simulink model "generic_IVS"  (R2024a)
settings: Solver=FixedStepDiscrete  StartTime=0.0  StopTime=inf  FixedStep=0.001  RelTol=1e-3
undefined symbols (not defined in the file): do_waypoints_tail_shifted_2, pathXY, route1_waypoint, route1_waypoint_raw, route2_waypoint, route2_waypoint_raw, route3_waypoint, route3_waypoint_raw, waypoints2
libraries: CarMaker4SL x431, slpidlib x19, dspsigops x3, simulink x1
(part 2 of 15)

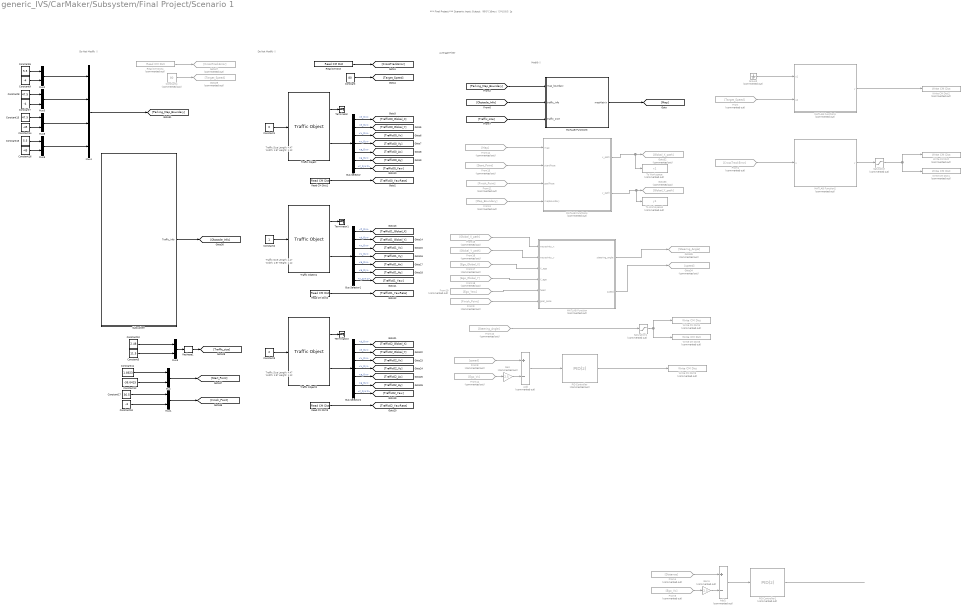
== system generic_IVS/CarMaker/Subsystem/Final Project/Scenario 1 ==
  note: Do Not Modify !!
  note: Traffic Size
      | Length: 4.47
      | Width: 1.97
      | Height: 1.12
  note: Traffic Size
      | Length: 4.47
      | Width: 1.97
      | Height: 1.12
  note: Traffic Size
      | Length: 4.47
      | Width: 1.97
      | Height: 1.12
  note: *** Final Project ***
      |
      | Scenario:
      | Input:
      | Output:
      | 제어기 10ms / 다익스트라 1s
  note: Do Not Modify !!
  note: Modify !!
  note: Average Filter
  Add : Sum  Commented=on  Inputs=+-
  Add1 : Sum  Commented=on  Inputs=+-
  Bus Selector : BusSelector  OutputSignals=t_0 x,t_0 y,v_0 x,v_0 y,a_0 x,a_0 y,r_zyx z
  Bus Selector1 : BusSelector  OutputSignals=t_0 x,t_0 y,v_0 x,v_0 y,a_0 x,a_0 y,r_zyx z
  Bus Selector2 : BusSelector  OutputSignals=t_0 x,t_0 y,v_0 x,v_0 y,a_0 x,a_0 y,r_zyx z
  Constant : Constant  Value=80
  Constant1 : Constant  Value=0
  Constant10 : Constant  Value=2.48
  Constant11 : Constant  Value=1.8923
  Constant12 : Constant  Value=-36.6415
  Constant13 : Constant  Value=47.5
  Constant14 : Constant  Value=-45
  Constant15 : Constant  Value=5.5
  Constant16 : Constant  Value=-45
  Constant17 : Constant  Value=36.5
  Constant18 : Constant  Value=-3
  Constant2 : Constant
  Constant3 : Constant  Value=2
  Constant4 : Constant  Commented=on  Value=80
  Constant5 : Constant  Value=11.5
  Constant6 : Constant  Value=5.5
  Constant7 : Constant  Value=-4
  Constant8 : Constant  Value=47.5
  Constant9 : Constant  Value=-4
  From : From  Commented=on  GotoTag=Target_Speed
  From1 : From  Commented=on  GotoTag=CrossTrackError
  From10 : From  Commented=on  GotoTag=Steering_Angle
  From11 : From  Commented=on  GotoTag=Finish_Point
  From12 : From  Commented=on  GotoTag=Map
  From13 : From  Commented=on  GotoTag=Start_Point
  From14 : From  Commented=on  GotoTag=Ego_Vx
  From15 : From  Commented=on  GotoTag=Global_X_path
  From16 : From  Commented=on  GotoTag=Global_Y_path
  From17 : From  Commented=on  GotoTag=Ego_Global_X
  From18 : From  Commented=on  GotoTag=Ego_Global_Y
  From19 : From  Commented=on  GotoTag=Ego_Yaw
  From3 : From  Commented=on  GotoTag=Map_Boundary
  From4 : From  Commented=on  GotoTag=Distance
  From5 : From  Commented=on  GotoTag=Ego_Vx
  From8 : From  Commented=on  GotoTag=speed
  From9 : From  Commented=on  GotoTag=Finish_Point
  Gain : Gain  Commented=on  Gain=2.5
  Gain1 : Gain  Commented=on  Gain=2.5
  Goto27 : Goto  Commented=on  GotoTag=CrossTrackError
  Goto29 : Goto  Commented=on  GotoTag=Target_Speed
  Goto32 : Goto  Commented=on  GotoTag=Global_X_path
  Goto33 : Goto  Commented=on  GotoTag=Global_Y_path
  Goto34 : Goto  Commented=on  GotoTag=speed
  Goto35 : Goto  Commented=on  GotoTag=Steering_Angle
  Ground : Ground  Commented=on
  MATLAB Function : MATLAB Function  Commented=on  TreatAsAtomicUnit=on
  MATLAB Function1 : MATLAB Function  Commented=on  TreatAsAtomicUnit=on
  MATLAB Function2 : MATLAB Function  Commented=on  TreatAsAtomicUnit=on
  MATLAB Function3 : MATLAB Function  TreatAsAtomicUnit=on
  MATLAB Function4 : MATLAB Function  Commented=on  TreatAsAtomicUnit=on
  Mux{,1..3,5,8..9} (7 alike) : Mux  Inputs=2
  Mux4 : Mux
  PID Controller : slpidlib/PID Controller  Commented=on  Controller=PID  Form=Parallel  TimeDomain=Discrete-time  UseExternalTs=off  SampleTime=-1  IntegratorMethod=Forward Euler  FilterMethod=Forward Euler  ControllerParametersSource=internal  P=1  I=0  UseKiTs=off  D=0  UseExternalDerivativeSource=off  N=100  UseFilter=off  TunerSelectOption=Transfer Function Based (PID Tuner App)  InitialConditionSource=internal  InitialConditionForIntegrator=0  InitialConditionForFilter=0  DifferentiatorICPrevScaledInput=0  ExternalReset=none  TrackingMode=off  Kt=1  LimitOutput=off  SatLimitsSource=internal  UpperSaturationLimit=inf  LowerSaturationLimit=-inf  LinearizeAsGain=on  AntiWindupMode=none  Kb=1  LimitIntegrator=off  UpperIntegratorSaturationLimit=inf  LowerIntegratorSaturationLimit=-inf  POutMin=[]  POutMax=[]  IOutMin=[]  IOutMax=[]  DOutMin=[]  DOutMax=[]  NOutMin=[]  NOutMax=[]  SumOutMin=[]  SumOutMax=[]  SaturationOutMin=[]  SaturationOutMax=[]  PParamMin=[]  PParamMax=[]  IParamMin=[]  IParamMax=[]  DParamMin=[]  DParamMax=[]  NParamMin=[]  NParamMax=[]  KbParamMin=[]  KbParamMax=[]  KtParamMin=[]  KtParamMax=[]  KbOutMin=[]  KbOutMax=[]  KtOutMin=[]  KtOutMax=[]  IntegratorOutMin=[]  IntegratorOutMax=[]  FilterOutMin=[]  FilterOutMax=[]  SumI1OutMin=[]  SumI1OutMax=[]  SumI2OutMin=[]  SumI2OutMax=[]  SumI3OutMin=[]  SumI3OutMax=[]  SumI4OutMin=[]  SumI4OutMax=[]  SumDOutMin=[]  SumDOutMax=[]  DifferentiatorOutMin=[]  DifferentiatorOutMax=[]  FilterDiffOutCoefMin=[]  FilterDiffOutCoefMax=[]  ReciprocalOutMin=[]  ReciprocalOutMax=[]  SumDenOutMin=[]  SumDenOutMax=[]  SumNumOutMin=[]  SumNumOutMax=[]  DivideOutMin=[]  DivideOutMax=[]  UdiffTsProdOutMin=[]  UdiffTsProdOutMax=[]  NTsProdOutMin=[]  NTsProdOutMax=[]  UintegralTsProdOutMin=[]  UintegralTsProdOutMax=[]  UngainTsProdOutMin=[]  UngainTsProdOutMax=[]  ClampingZeroOutDataTypeStr=Inherit: Inherit via back propagation  ClampingZeroOutMin=[]  ClampingZeroOutMax=[]  FilterDenConstantOutDataTypeStr=Inherit: Inherit via back propagation  FilterDenConstantOutMin=[]  FilterDenConstantOutMax=[]  PCopyOutDataTypeStr=Inherit: Inherit via back propagation  PCopyOutMin=[]  PCopyOutMax=[]  NCopyOutDataTypeStr=Inherit: Inherit via back propagation  NCopyOutMin=[]  NCopyOutMax=[]  IntegratorContinuousStateAttributes=''  IntegratorStateMustResolveToSignalObject=off  IntegratorRTWStateStorageClass=Auto  FilterContinuousStateAttributes=''  FilterStateMustResolveToSignalObject=off  FilterRTWStateStorageClass=Auto  ParallelPVariant=InternalParameters  IdealPVariant=Disabled  IVariant=InternalParameters  DVariant=InternalParameters  IntegratorVariant=Discrete  SatVariant=Disabled  AWVariant=Passthrough  PCopyVariant=Disabled  TRVariant=Disabled  FdbkBlocksVariant=Forward  IdealPFdbkVariant=Disabled  SatFdbkVariant=Disabled  DerivativeFilterVariant=Differentiator  NVariant=Passthrough  NCopyVariant=Disabled_SignalSpec  FilterICVariant=InternalICsDifferentiator  IntegratorICVariant=InternalICs  ExternalResetVariant=Disabled  TRSumVariant=Passthrough  SumFdbkVariant=Disabled  SumVariant=Sum_PID  TsampFilterVariant=InternalTs  TsampNgainVariant=Passthrough  TsampIntegralVariant=Disabled_SignalSpec  ExternalSaturationOutDataTypeStr=Inherit: Same as second input  DerivativeSourceVariant=ErrorSignal
  PID Controller1 : slpidlib/PID Controller  Commented=on  Controller=PID  Form=Parallel  TimeDomain=Discrete-time  UseExternalTs=off  SampleTime=-1  IntegratorMethod=Forward Euler  FilterMethod=Forward Euler  ControllerParametersSource=internal  P=5  I=0  UseKiTs=off  D=0  UseExternalDerivativeSource=off  N=100  UseFilter=off  TunerSelectOption=Transfer Function Based (PID Tuner App)  InitialConditionSource=internal  InitialConditionForIntegrator=0  InitialConditionForFilter=0  DifferentiatorICPrevScaledInput=0  ExternalReset=none  TrackingMode=off  Kt=1  LimitOutput=off  SatLimitsSource=internal  UpperSaturationLimit=inf  LowerSaturationLimit=-inf  LinearizeAsGain=on  AntiWindupMode=none  Kb=1  LimitIntegrator=off  UpperIntegratorSaturationLimit=inf  LowerIntegratorSaturationLimit=-inf  POutMin=[]  POutMax=[]  IOutMin=[]  IOutMax=[]  DOutMin=[]  DOutMax=[]  NOutMin=[]  NOutMax=[]  SumOutMin=[]  SumOutMax=[]  SaturationOutMin=[]  SaturationOutMax=[]  PParamMin=[]  PParamMax=[]  IParamMin=[]  IParamMax=[]  DParamMin=[]  DParamMax=[]  NParamMin=[]  NParamMax=[]  KbParamMin=[]  KbParamMax=[]  KtParamMin=[]  KtParamMax=[]  KbOutMin=[]  KbOutMax=[]  KtOutMin=[]  KtOutMax=[]  IntegratorOutMin=[]  IntegratorOutMax=[]  FilterOutMin=[]  FilterOutMax=[]  SumI1OutMin=[]  SumI1OutMax=[]  SumI2OutMin=[]  SumI2OutMax=[]  SumI3OutMin=[]  SumI3OutMax=[]  SumI4OutMin=[]  SumI4OutMax=[]  SumDOutMin=[]  SumDOutMax=[]  DifferentiatorOutMin=[]  DifferentiatorOutMax=[]  FilterDiffOutCoefMin=[]  FilterDiffOutCoefMax=[]  ReciprocalOutMin=[]  ReciprocalOutMax=[]  SumDenOutMin=[]  SumDenOutMax=[]  SumNumOutMin=[]  SumNumOutMax=[]  DivideOutMin=[]  DivideOutMax=[]  UdiffTsProdOutMin=[]  UdiffTsProdOutMax=[]  NTsProdOutMin=[]  NTsProdOutMax=[]  UintegralTsProdOutMin=[]  UintegralTsProdOutMax=[]  UngainTsProdOutMin=[]  UngainTsProdOutMax=[]  ClampingZeroOutDataTypeStr=Inherit: Inherit via back propagation  ClampingZeroOutMin=[]  ClampingZeroOutMax=[]  FilterDenConstantOutDataTypeStr=Inherit: Inherit via back propagation  FilterDenConstantOutMin=[]  FilterDenConstantOutMax=[]  PCopyOutDataTypeStr=Inherit: Inherit via back propagation  PCopyOutMin=[]  PCopyOutMax=[]  NCopyOutDataTypeStr=Inherit: Inherit via back propagation  NCopyOutMin=[]  NCopyOutMax=[]  IntegratorContinuousStateAttributes=''  IntegratorStateMustResolveToSignalObject=off  IntegratorRTWStateStorageClass=Auto  FilterContinuousStateAttributes=''  FilterStateMustResolveToSignalObject=off  FilterRTWStateStorageClass=Auto  ParallelPVariant=InternalParameters  IdealPVariant=Disabled  IVariant=InternalParameters  DVariant=InternalParameters  IntegratorVariant=Discrete  SatVariant=Disabled  AWVariant=Passthrough  PCopyVariant=Disabled  TRVariant=Disabled  FdbkBlocksVariant=Forward  IdealPFdbkVariant=Disabled  SatFdbkVariant=Disabled  DerivativeFilterVariant=Differentiator  NVariant=Passthrough  NCopyVariant=Disabled_SignalSpec  FilterICVariant=InternalICsDifferentiator  IntegratorICVariant=InternalICs  ExternalResetVariant=Disabled  TRSumVariant=Passthrough  SumFdbkVariant=Disabled  SumVariant=Sum_PID  TsampFilterVariant=InternalTs  TsampNgainVariant=Passthrough  TsampIntegralVariant=Disabled_SignalSpec  ExternalSaturationOutDataTypeStr=Inherit: Same as second input  DerivativeSourceVariant=ErrorSignal
  Read CM Dict : CarMaker4SL/Read CM Dict  xname=Car.Road.Path.DevDist  xsync=off  xstime=Inherited
  Read CM Dict1 : CarMaker4SL/Read CM Dict  xname=Traffic.T22.rzv  xsync=off  xstime=Inherited
  Read CM Dict2 : CarMaker4SL/Read CM Dict  xname=Traffic.T23.rzv  xsync=off  xstime=Inherited
  Read CM Dict3 : CarMaker4SL/Read CM Dict  xname=Traffic.T24.rzv  xsync=off  xstime=Inherited
  Read CM Dict4 : CarMaker4SL/Read CM Dict  Commented=on  xname=Car.Road.Path.DevDist  xsync=off  xstime=Inherited
  Reshape1 : Reshape  OutputDimensionality=Row vector (2-D)  OutputDimensions=[2,2]
  Saturation : Saturate  Commented=on  UpperLimit=2  LowerLimit=-2
  Saturation1 : Saturate  Commented=on  UpperLimit=pi/6  LowerLimit=-pi/6
  Subsystem : Subsystem
  Terminator : Terminator
  Terminator1 : Terminator
  Terminator2 : Terminator
  To Workspace : ToWorkspace  Commented=on  VariableName=x1  SaveFormat=Timeseries  SampleTime=-1
  To Workspace1 : ToWorkspace  Commented=on  VariableName=y1  SaveFormat=Timeseries  SampleTime=-1
  Traffic Object : CarMaker4SL/Traffic Object  xname=T00  ximode=Traffic Id  xstime=Inherited
      settings: SourceProductName=CarMaker4SL
  Traffic Object1 : CarMaker4SL/Traffic Object  xname=T01  ximode=Traffic Id  xstime=Inherited
      settings: SourceProductName=CarMaker4SL
  Traffic Object2 : CarMaker4SL/Traffic Object  xname=T02  ximode=Traffic Id  xstime=Inherited
      settings: SourceProductName=CarMaker4SL
  Write CM Dict : CarMaker4SL/Write CM Dict  Commented=on  xname=Car.CFL.rz_ext  xsync=off
  Write CM Dict1 : CarMaker4SL/Write CM Dict  Commented=on  xname=Car.CFR.rz_ext  xsync=off
  Write CM Dict2 : CarMaker4SL/Write CM Dict  Commented=on  xname=AccelCtrl.DesiredAx  xsync=off
  Write CM Dict3 : CarMaker4SL/Write CM Dict  Commented=on  xname=AccelCtrl.DesiredAx  xsync=off
  Write CM Dict4 : CarMaker4SL/Write CM Dict  Commented=on  xname=Car.CFL.rz_ext  xsync=off
  Write CM Dict5 : CarMaker4SL/Write CM Dict  Commented=on  xname=Car.CFR.rz_ext  xsync=off
  wires:
  Saturation/1 -> Write CM Dict/1, Write CM Dict1/1
  Constant1/1 -> Traffic Object/1
  MATLAB Function2/1(y) -> Saturation/1
  MATLAB Function1/1(y) -> Write CM Dict2/1
  From1/1 -> MATLAB Function2/1(u)
  Ground/1 -> MATLAB Function1/1(u1)
  Read CM Dict/1 -> [CrossTrackError]
  From/1 -> MATLAB Function1/2(u2)
  Constant/1 -> [Target_Speed]
  Bus Selector/4 -> [Traffic00_Vy]  "<v_0 y>"
  Traffic Object/1 -> Terminator/1
  Bus Selector/3 -> [Traffic00_Vx]  "<v_0 x>"
  Traffic Object/2 -> Bus Selector/1
  Bus Selector/1 -> [Traffic00_Global_X]  "<t_0 x>"
  Bus Selector/2 -> [Traffic00_Global_Y]  "<t_0 y>"
  Read CM Dict1/1 -> [Traffic00_YawRate]
  Bus Selector/5 -> [Traffic00_Ax]  "<a_0 x>"
  Bus Selector/6 -> [Traffic00_Ay]  "<a_0 y>"
  Bus Selector/7 -> [Traffic00_Yaw]  "<r_zyx z>"
  Read CM Dict2/1 -> [Traffic01_YawRate]
  Bus Selector1/1 -> [Traffic01_Global_X]  "<t_0 x>"
  Bus Selector1/5 -> [Traffic01_Ax]  "<a_0 x>"
  Bus Selector1/6 -> [Traffic01_Ay]  "<a_0 y>"
  Bus Selector1/7 -> [Traffic01_Yaw]  "<r_zyx z>"
  Traffic Object1/1 -> Terminator1/1
  Bus Selector1/4 -> [Traffic01_Vy]  "<v_0 y>"
  Constant2/1 -> Traffic Object1/1
  Traffic Object1/2 -> Bus Selector1/1
  Bus Selector1/3 -> [Traffic01_Vx]  "<v_0 x>"
  Bus Selector1/2 -> [Traffic01_Global_Y]  "<t_0 y>"
  Bus Selector2/3 -> [Traffic02_Vx]  "<v_0 x>"
  Bus Selector2/2 -> [Traffic02_Global_Y]  "<t_0 y>"
  Traffic Object2/2 -> Bus Selector2/1
  Bus Selector2/1 -> [Traffic02_Global_X]  "<t_0 x>"
  Bus Selector2/6 -> [Traffic02_Ay]  "<a_0 y>"
  Constant3/1 -> Traffic Object2/1
  Traffic Object2/1 -> Terminator2/1
  Bus Selector2/7 -> [Traffic02_Yaw]  "<r_zyx z>"
  Bus Selector2/5 -> [Traffic02_Ax]  "<a_0 x>"
  Read CM Dict3/1 -> [Traffic02_YawRate]
  Bus Selector2/4 -> [Traffic02_Vy]  "<v_0 y>"
  Constant10/1 -> Mux3/1
  Constant5/1 -> Mux3/2
  Reshape1/1 -> [Traffic_size]
  Mux3/1 -> Reshape1/1
  Read CM Dict4/1 -> Goto27/1
  Constant4/1 -> Goto29/1
  Constant16/1 -> Mux9/2
  Mux4/1 -> [Parking_Map_Boundary]
  Constant14/1 -> Mux8/2
  Mux9/1 -> Mux4/4
  Constant9/1 -> Mux2/2
  Mux5/1 -> Mux4/2
  Constant7/1 -> Mux5/2
  Mux8/1 -> Mux4/3
  Mux2/1 -> Mux4/1
  Constant6/1 -> Mux2/1
  Constant13/1 -> Mux8/1
  Constant15/1 -> Mux9/1
  Constant8/1 -> Mux5/1
  Subsystem/1(Traffic_Info) -> [Obstacle_Info]
  Gain/1 -> Add/2
  From11/1 -> MATLAB Function4/3(goalPose)
  From9/1 -> MATLAB Function/6(goal_pose)
  MATLAB Function/2(speed) -> Goto34/1
  From18/1 -> MATLAB Function/4(Y_ego)
  From3/1 -> MATLAB Function4/4(mapboundary)
  From14/1 -> Gain/1
  Add1/1 -> PID Controller1/1
  From4/1 -> Add1/1
  Gain1/1 -> Add1/2
  From5/1 -> Gain1/1
  From16/1 -> MATLAB Function/2(waypoints_y)
  [Parking_Map_Boundary] -> MATLAB Function3/1(map_boundary)
  PID Controller1/1 -> ?
  From8/1 -> Add/1
  PID Controller/1 -> Write CM Dict3/1
  MATLAB Function4/2(y_path) -> To Workspace1/1, Goto33/1
  From19/1 -> MATLAB Function/5(head)
  From10/1 -> Saturation1/1
  From17/1 -> MATLAB Function/3(X_ego)
  [Traffic_size] -> MATLAB Function3/3(traffic_size)
  From12/1 -> MATLAB Function4/1(map)
  Saturation1/1 -> Write CM Dict4/1, Write CM Dict5/1
  MATLAB Function3/1(mapMatrix) -> [Map]
  MATLAB Function4/1(x_path) -> To Workspace/1, Goto32/1
  [Obstacle_Info] -> MATLAB Function3/2(traffic_info)
  From13/1 -> MATLAB Function4/2(startPose)
  Add/1 -> PID Controller/1
  MATLAB Function/1(steering_angle) -> Goto35/1
  From15/1 -> MATLAB Function/1(waypoints_x)
  Constant17/1 -> Mux1/1
  Constant12/1 -> Mux/2
  Constant18/1 -> Mux1/2
  Mux1/1 -> [Finish_Point]
  Constant11/1 -> Mux/1
  Mux/1 -> [Start_Point]
